simulink model "my_robot_sim"  (R2020a)
settings: Solver=VariableStepAuto  StartTime=0.0  StopTime=10  RelTol=1e-3
libraries: roblocks x3
settings Model: Creator=rusta  LastModifiedBy=rusta

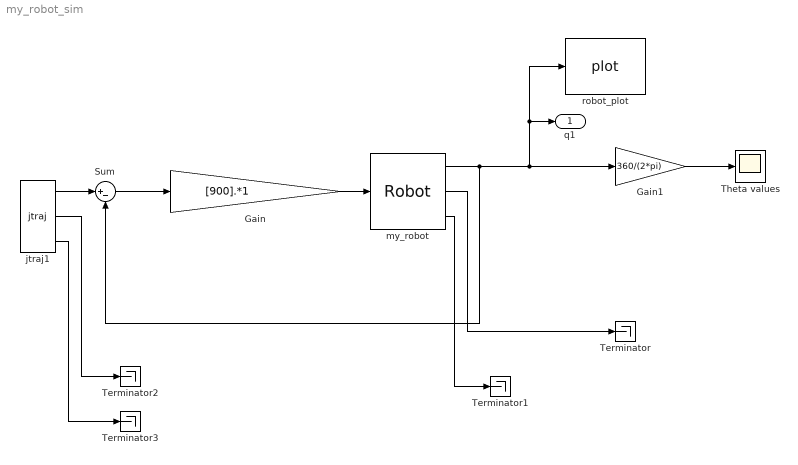
== system my_robot_sim ==
  Gain : Gain  Gain=[900].*1
  Gain1 : Gain  Gain=360/(2*pi)
  Sum : Sum  Inputs=|+-
  Terminator{,1..3} (4 alike) : Terminator
  Theta values : Scope
  jtraj1 : roblocks/Toolbox/jtraj  q0=[0 0 0]  qf=[pi/2 -pi/4 -pi/4]  tmax=2  ts=0.02
  my_robot : roblocks/Arm/Robot  robot=rrr  q0=[0 0 0]
  robot_plot : roblocks/Arm/plot  robot=rrr  fps=5  holdplot=on
  q1 : Outport
  wires:
  jtraj1/1 -> Sum/1
  Sum/1 -> Gain/1
  Gain1/1 -> Theta values/1
  Gain/1 -> my_robot/1
  my_robot/1 -> Sum/2, Gain1/1, q1/1, robot_plot/1
  my_robot/2 -> Terminator/1
  my_robot/3 -> Terminator1/1
  jtraj1/2 -> Terminator2/1
  jtraj1/3 -> Terminator3/1
